simulink model "HQEV_MiL_20160830_integrate"  (Simulink 8.3)
settings: Solver=FixedStepDiscrete  StartTime=0.0  StopTime=inf  FixedStep=0.01  RelTol=1e-3
PostLoadFcn:
  | , if any(exist('dsrtsu_mdlpostloadfcn', 'file') == [2, 3, 6]), try dsrtsu_mdlpostloadfcn('Execute', bdroot); catch fprintf('Error in PostLoadFcn (dsrtsu_mdlpostloadfcn) for model "%s":\n %s\n', bdroot, lasterr); end, end,
values from neighbouring files (symbols this model uses):
  Bat_C_Ah = 36    [parameter_V1.mat]
  Bat_ocv_xIndex = [5 10 20 30 40 50 60 70 80 90 95]    [parameter_V1.mat]
  Bat_ocv_z = [329 332 340 345 347 351 358 372 377 386 391]    [parameter_V1.mat]
  Bat_R_ohm_z = [4.41 3.46 1.57 1.07 0.76 0.63 0.55 0.44 0.41 0.4 0.4 3.14 ... (66 elements, 11x6)]    [parameter_V1.mat]
  Bat_SOC_Init = 90    [parameter_V1.mat]
  Env_hum_pct_Ambient = 30    [parameter_V1.mat]
  Env_Slope_deg = 0    [parameter_V1.mat]
  Env_Temp_degC_Ambient = 25    [parameter_V1.mat]
  Env_v_kmph_HWind = 0    [parameter_V1.mat]
  Reducer_F_i = 7.23    [parameter_V1.mat]
  Reducer_R_i = 7.23    [parameter_V1.mat]
  Veh =     [parameter_V1.mat]
  Veh_A_m2_Fr = 2.246    [parameter_V1.mat]
  Veh_F_Brake =     [parameter_V1.mat]
  Veh_fac_AirDrag = 0.326    [parameter_V1.mat]
  Veh_fac_WhDragFrict_0 = 0.011    [parameter_V1.mat]
  Veh_g_mps2_C = 9.81    [parameter_V1.mat]
  Veh_GainBrake =     [parameter_V1.mat]
  Veh_h_m_COGHigh = 0.5    [parameter_V1.mat]
  Veh_J_kgm2_Wh = 1.3635    [parameter_V1.mat]
  Veh_L_m_AxlBas = 2.63    [parameter_V1.mat]
  Veh_M_kg = 1427    [parameter_V1.mat]
  Veh_mu_Brake = 0.4    [parameter_V1.mat]
  Veh_mu_Tyre =     [parameter_V1.mat]
  Veh_num_FrictPair = 8    [parameter_V1.mat]
  Veh_pct_Brk = 70    [parameter_V1.mat]
  Veh_r_dyn =     [parameter_V1.mat]
  Veh_r_m_BrkDisk = 0.136    [parameter_V1.mat]
  Veh_rho_kgpm3_Air = 1.2258    [parameter_V1.mat]
undefined symbols (not defined in the file or in its folder): DiscIntNeverNeededParam, p_bool_False_M, p_bool_True_M
libraries: BaseOperationLib_Browser x38, simulink x9, DTQC_lib x1, ERR_lib x1, MQM_lib x1, PTCL_lib x1, PUD_lib x1, TQD_lib x1, TQR_lib x1, VMM_lib x1, ACCA_lib x1, BBCA_lib x1
(part 3 of 15)

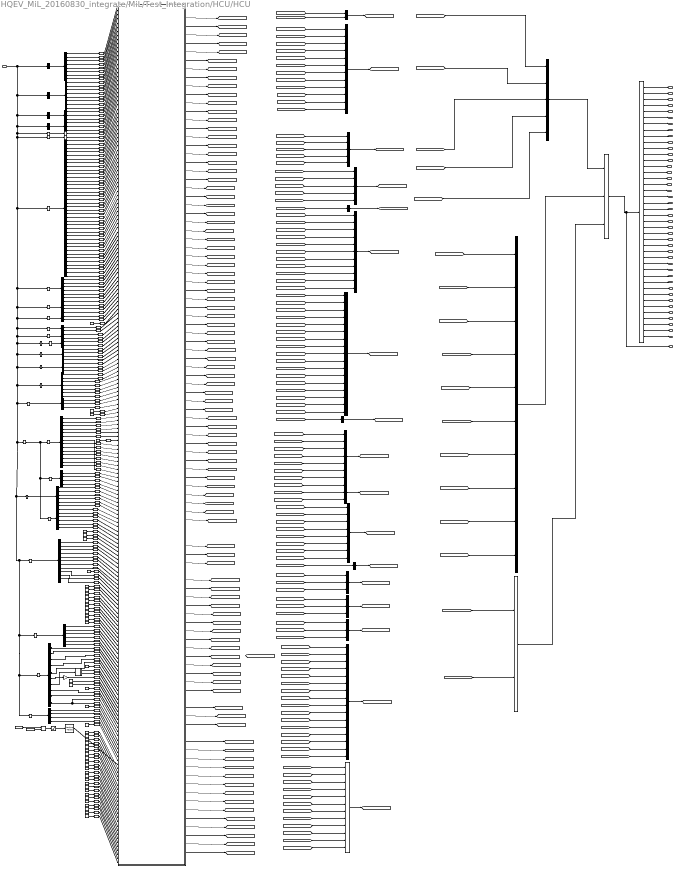
== system HQEV_MiL_20160830_integrate/MiL/Test_Integration/HCU/HCU ==
  In1 : Inport
  AccPedpct2mV : Subsystem
  Bus Creator : BusCreator  Inputs=12
  Bus Creator1 : BusCreator  Inputs=5
  Bus Creator10 : BusCreator  Inputs=8
  Bus Creator11 : BusCreator  Inputs=1
  Bus Creator12 : BusCreator  Inputs=16
  Bus Creator13 : BusCreator  Inputs=12
  Bus Creator{9,14..16,20} (5 alike) : BusCreator  Inputs=3
  Bus Creator17 : BusCreator  Inputs=5
  Bus Creator18 : BusCreator  Inputs=10
  Bus Creator19 : BusCreator  Inputs=2
  Bus Creator2 : BusCreator  Inputs=5
  Bus Creator3 : BusCreator  Inputs=1
  Bus Creator4 : BusCreator  Inputs=2
  Bus Creator5 : BusCreator  Inputs=11
  Bus Creator6 : BusCreator  Inputs=17
  Bus Creator7 : BusCreator  Inputs=1
  Bus Creator8 : BusCreator  Inputs=7
  Bus Selector : BusSelector  OutputSignals=HCU_EVCAN.EV_ACU_1.pOUTP_st_ACU1Crash,HCU_EVCAN.EV_HCU_2.pOUTP_V_HCU2DCDCOutVoltReq,HCU_EVCAN.EV_HCU_2.pOUTP_bool_HCU2DCDCEnbl,HCU_EVCAN.EV_HCU_2.pOUTP_bool_HCU2MainPlusCtrl,HCU_EVCAN.EV_HCU_2.pOUTP_bool_HCU2MainMinusCtrl,HCU_EVCAN.EV_HCU_2.pOUTP_bool_HCU2PreChrgCtrl,HCU_EVCAN.EV_HCU_2.pOUTP_bool_HCU2ChrgPlusCtrl,HCU_EVCAN.EV_HCU_2.pOUTP_bool_HCU2ChrgMinusCtrl,HCU_EVCAN.EV_HCU_2.pOUTP_bool_HCU2SleepIndSig,HCU_EVCAN.EV_HCU_2.pOUTP_st_HCU2ChrgHeatPms,HCU_EVCAN.EV_HCU_2.pOUTP_st_HCU2ChrgConnSt,HCU_EVCAN.EV_HCU_2.pOUTP_bool_HCU2ChrgPms,HCU_EVCAN.EV_HCU_2.pOUTP_st_HCU2VehOprtMode,HCU_EVCAN.EV_HCU_3.pOUTP_Nm_HCU3TMTorqReqToMCU1,HCU_EVCAN.EV_HCU_3.pOUTP_bool_HCU3MotCtlrStModReqToMCU1,HCU_EVCAN.EV_HCU_3.pOUTP_bool_HCU3StopReqToMCU1,HCU_EVCAN.EV_HCU_3.pOUTP_bool_HCU3MotRpdDchaReqToMCU1,HCU_EVCAN.EV_HCU_3.pOUTP_bool_HCU3AntijerkOffReqToMCU1,HCU_EVCAN.EV_HCU_5.pOUTP_Nm_HCU5TMToqReqToMCU2,HCU_EVCAN.EV_HCU_5.pOUTP_bool_HCU5MotCtlrStModReqToMCU2,HCU_EVCAN.EV_HCU_5.pOUTP_bool_HCU5StopReqToMCU2,HCU_EVCAN.EV_HCU_5.pOUTP_bool_HCU5MotRpdDchaReqToMCU2,HCU_EVCAN.EV_HCU_5.pOUTP_bool_HCU5AntijerkOffReqToMCU2,HCU_PTCAN.PT_HCU_13.HCU_VehicleDeiceHeatPermit,HCU_PTCAN.PT_HCU_13.pOUTP_st_HCU13BatPackCoolReq,HCU_PTCAN.PT_HCU_13.pOUTP_bool_HCU13IGOffReq,HCU_PTCAN.PT_HCU_13.HCU_BatterySOCWarning,HCU_PTCAN.PT_HCU_5.pOUTP_st_HCU5EVReady,HCU_PTCAN.PT_HCU_5.pOUTP_st_HCU5HCUStatus,HCU_PTCAN.HCU_Epark.HCU_ParkRequest,HCU_IO.HCU_IO_OUT.pOUTP_pwm_PTCPWMCtrl,HCU_IO.HCU_IO_OUT.pOUTP_bool_LoCoolFanRlyCtrl,HCU_IO.HCU_IO_OUT.pOUTP_bool_HiCoolFanRlyCtrl,HCU_IO.HCU_IO_OUT.pOUTP_pwm_MotWaterPump1Ctrl,HCU_IO.HCU_IO_OUT.pOUTP_pwm_MotWaterPump2Ctrl,HCU_IO.HCU_IO_OUT.pOUTP_pwm_BatWaterPumpCtrl,HCU_PTCAN.PT_HCU_14.HCU_LeverInfo,HCU_PTCAN.PT_HCU_15,HCU_PTCAN.PT_HCU_18,HCU_PTCAN.PT_HCU_19,HCU_PTCAN.PT_HCU_4,HCU_PTCAN.PT_HCU_8
  Bus Selector1 : BusSelector  OutputSignals=MCU_F
  Bus Selector10 : BusSelector  OutputSignals=MCU_F
  Bus Selector11 : BusSelector  OutputSignals=MCU_R
  Bus Selector12 : BusSelector  OutputSignals=MCU2_CoolingRequest
  Bus Selector13 : BusSelector  OutputSignals=BMS
  Bus Selector14 : BusSelector  OutputSignals=BMS_BatteryPackVoltage,BMS_BatteryPackCurrent,BMS_FaultDisposeSignal,BMS_MainPlusContactorCoilState,BMS_MainMinusContactorCoilState,BMS_PrechargeContactorCoilState,BMS_ChargePlusContactorCoilState,BMS_ChargeMinusContactorCoilState,BMS_MainMinusContactorCoilFault,BMS_PrechargeContactorCoilFault,BMS_ChargePlusContactorCoilFault,BMS_ChargeMinusContactorCoilFault,BMS_MainPlusContactorFault,BMS_ChargeRequest,BMS_ChargeStatus,BMS_MainPlusContactorCoilFault,BMS_ChargePlusContactorFault,BMS_BatteryPackStatus,BMS_BatteryChargePowerAvailable_10,BMS_BatteryDischargePowerAvailable_10,BMS_BatteryChargePowerAvailable_2,BMS_BatteryDischargePowerAvailable_2,BMS_BatteryPackSOH,BMS_BatteryPackTemperature,BMS_BatteryPackSOC,BMS_HeatingRequest,BMS_BatteryPackMAXTemperature,BMS_BatteryPackMINTemperature,BMS_BatteryPackInletWaterTemperature,BMS_RemainingEnergyRatio,BMS_ChargeStationOutputCurrent,BMS_ChargeStationOutputVoltage,BMS_InstantPowerConsumption,BMS_ChargeStationStatus,BMS_ChargeStationParameterConfigStatus,BMS_InsulationMonitorWarning,BMS_RemainingChargeTime,BMS_ChargeStationHandShakeStatus
  Bus Selector15 : BusSelector  OutputSignals=DCDC
  Bus Selector16 : BusSelector  OutputSignals=DCDC_OutputCurrent,DCDC_Status,DCDC_OutputVoltage,DCDC_InputCurrent,DCDC_Temperature,DCDC_InputVoltage
  Bus Selector17 : BusSelector  OutputSignals=Charger
  Bus Selector18 : BusSelector  OutputSignals=Charger_Status,Charger_Temperature,Charger_OutputVoltage,Charger_RechargeRequest
  Bus Selector19 : BusSelector  OutputSignals=Airbag
  Bus Selector2 : BusSelector  OutputSignals=MCU1_TMSpeed,MCU1_ActTMTorque,MCU1_TMCapacitanceVoltage,MCU1_ActualTMTorqueValid,MCU1_PrechargeAllow,MCU1_TMStatus,MCU1_TMErrorStatus,MCU1_ShutdownEnable
  Bus Selector20 : BusSelector  OutputSignals=ACU_Crash,ACU_ErrorStatus
  Bus Selector21 : BusSelector  OutputSignals=EPS
  Bus Selector22 : BusSelector  OutputSignals=EPSErrorStatus,SteeringWheelAngleStatus
  Bus Selector23 : BusSelector  OutputSignals=IC
  Bus Selector24 : BusSelector  OutputSignals=HandBrakeSt,DDSPS
  Bus Selector25 : BusSelector  OutputSignals=ESP
  Bus Selector26 : BusSelector  OutputSignals=EPB
  Bus Selector27 : BusSelector  OutputSignals=EPB_Status,EPB_ErrorStatus
  Bus Selector28 : BusSelector  OutputSignals=Epark
  Bus Selector29 : BusSelector  OutputSignals=ParkLock,ParkSensor,DriveSensor,ePARK_CAN_ERR
  Bus Selector3 : BusSelector  OutputSignals=MCU2_TMSpeed,MCU2_ActTMTorque,MCU2_TMCapacitanceVoltage,MCU2_ActualTMTorqueValid,MCU2_PrechargeAllow,MCU2_TMStatus,MCU2_TMErrorStatus,MCUShutdownEnable
  Bus Selector30 : BusSelector  OutputSignals=BCM
  Bus Selector31 : BusSelector  OutputSignals=DriverDoorSt,BCM_HighBeamCmd,WiperStatus
  Bus Selector32 : BusSelector  OutputSignals=Drv
  Bus Selector33 : BusSelector  OutputSignals=signal2.ParkButton (signal 11),signal2.EGSM_ECOSButton (signal 14),signal2.Lever_Position (signal 1)
  Bus Selector34 : BusSelector  OutputSignals=EBS
  Bus Selector35 : BusSelector  OutputSignals=SOC,T_BATT,Status_Temp,ERROR_Calib,Resp_Error,FLAG_INCONSISTENCY,SOC_STATE
  Bus Selector36 : BusSelector  OutputSignals=ESP
  Bus Selector37 : BusSelector  OutputSignals=WheelSpeed_FL,WheelSpeed_FR,ABS_VehicleSpeed,WheelSpeed_RL,WheelSpeed_RR,ABS_MasterCylinderPressure,ABS_ErrorStatus,ABS_Intervention,ASR_ErrorStatus,ASR_Intervention,ESP_ErrorStatus,ESP_Intervention,HHC_Status,HHC_Available
  Bus Selector38 : BusSelector  OutputSignals=ABS
  Bus Selector39 : BusSelector  OutputSignals=YRS
  Bus Selector4 : BusSelector  OutputSignals=MCU_R
  Bus Selector40 : BusSelector  OutputSignals=AX1,AY1,YRSStatus,YRSErrorStatus,AX1Offset,AY1Offset
  Bus Selector41 : BusSelector  OutputSignals=ASR
  Bus Selector42 : BusSelector  OutputSignals=ASR_TorqueReductionFast,MSR_TorqueIncrease,ASR_StatusTRFast,MSR_StatusTI
  Bus Selector43 : BusSelector  OutputSignals=AC
  Bus Selector44 : BusSelector  OutputSignals=AC_CompressorOnRequest,AC_Status,AC_FanRequest,AC_PTCStatus,AC_shutdownEnableL,AC_PowerConsumptionL,AC_PowerConsumptionH,AC_ShutdownEnableH,ACIndication,AC_BLWLevelIndication,AC_OutsideTemperatureIndication
  Bus Selector45 : BusSelector  OutputSignals=ACC
  Bus Selector46 : BusSelector  OutputSignals=ACC_ErrorStatus,ACC_Status,ACC_DecelerationRequest,ACC_StatusTorqueRequest,ACC_TorqueRequest,ACC_StatusACCDecelerationRequest
  Bus Selector47 : BusSelector  OutputSignals=Drv
  Bus Selector48 : BusSelector  OutputSignals=signal2.FastCharge (signal 6),signal2.FastCharge (signal 7),signal2.interlockA (signal 2),signal2.InterlockB (signal 3),signal2.ACC_CruiseButton (signal 16),signal1.AccPed_pct,signal1.BrkPed_pct,signal2.KeyONState (signal 4),signal2.KeyStartState (signal 5),signal1.Brake_OnOff
  Bus Selector49 : BusSelector  OutputSignals=IO
  Bus Selector5 : BusSelector  OutputSignals=MCU1_TM_MAMTorque,MCU1_TM_MAGTorque,MCU1_CalTMTorque
  Bus Selector50 : BusSelector  OutputSignals=SlowChrgSensr1Temp,FastChrgSensr1Temp,SlowChrgSensr2Temp,FastChrgSensr2Temp
  Bus Selector51 : BusSelector  OutputSignals=ESP
  Bus Selector52 : BusSelector  OutputSignals=ASR2.ASR2TrqRdctFastASR2,ASR2.ASR2TrqIncrsMSR2,ASR2.ASR2StTRFastASR2,ASR2.ASR2StTIMSR2,ASR2.ABS6RegenTrqReq,ASR2.ABS6StRegenTrqReq
  Bus Selector6 : BusSelector  OutputSignals=MCU_F
  Bus Selector7 : BusSelector  OutputSignals=MCU_R
  Bus Selector8 : BusSelector  OutputSignals=MCU2_TM_MAMTorque,MCU2_TM_MAGTorque,MCU2_CalTMTorque
  Bus Selector9 : BusSelector  OutputSignals=MCU1_CoolingRequest
  Constant{1..4,6..22,48..68,70,76..77,80} (46 alike) : Constant  Value=0
  Constant23 : Constant  Value=101.325
  Constant24 : Constant
  Constant5 : Constant  Value=2
  Constant73 : Constant  Value=14
  Constant85 : Constant  Value=2
  Data Type Conversion{,1..44,60..80,82,85..105,107..158,160..162,164..167,169..172,177..229,237..241} (209 alike) : DataTypeConversion
  Gain : Gain  Gain=2
  HCU : Subsystem
  Lookup Table : BaseOperationLib_Browser/Lookup Tables Changed/Lookup Table  InputValues=[44.8 44.9 110.2 110.3]  Table=[0 500 4500 4600]  LookUpMeth=Interpolation-Use End Values  OutMin=[]  OutMax=[]  OutDataType=fixdt(1, 16)  OutScaling=2^0  OutDataTypeStr=Inherit: Inherit via back propagation  SaturateOnIntegerOverflow=on
      settings: AttributesFormatString=X:%<InputValues>\nTAB:%<Table>
  Product : Product  RndMeth=Zero
  Saturation : Saturate  UpperLimit=110.3  LowerLimit=44.8
  ACU_Crash : Outport
  HCU_DCDCOutputVoltageRequest : Outport  Port=2
  HCU_DCDCEnable : Outport  Port=3
  HCU_MainPosContactorControl : Outport  Port=4
  HCU_MainNegContactorControl : Outport  Port=5
  HCU_PrechargeContactorControl : Outport  Port=6
  HCU_ChargePosContactorControl : Outport  Port=7
  HCU_ChargeNegContactorControl : Outport  Port=8
  HCU_SleepIndication : Outport  Port=9
  HCU_ChargeHeatingPermission : Outport  Port=10
  HCU_ChargeConnectStatus : Outport  Port=11
  HCU_ChargePermission : Outport  Port=12
  HCU_VehicleOperatingMode : Outport  Port=13
  HCU_TMTorqueRequestToMCU1 : Outport  Port=14
  HCU_StatusTMRequestToMCU1 : Outport  Port=15
  HCU_StopRequestToMCU1 : Outport  Port=16
  HCU_RapidDischargeCmdToMCU1 : Outport  Port=17
  HCU_AntiJerkDisableCmdToMCU1 : Outport  Port=18
  HCU_TMTorqueRequestToMCU2 : Outport  Port=19
  HCU_StatusTMRequestToMCU2 : Outport  Port=20
  HCU_StopRequestToMCU2 : Outport  Port=21
  HCU_RapidDischargeCmdToMCU2 : Outport  Port=22
  HCU_AntiJerkDisableCmdToMCU2 : Outport  Port=23
  HCU_VehicleDeiceHeatPermit : Outport  Port=24
  HCU_BatteryPackCoolRequest : Outport  Port=25
  HCU_IGOFFRequest : Outport  Port=26
  HCU_BatterySOCWarning : Outport  Port=27
  HCU_EVReady : Outport  Port=28
  HCU_Status : Outport  Port=29
  HCU_ParkRequest : Outport  Port=30
  PTC_PWM_pct : Outport  Port=31
  LowSpdFanCmd_na : Outport  Port=32
  HighSpdFanCmd_na : Outport  Port=33
  EM1PumpCmd_pct : Outport  Port=34
  EM2PumpCmd_pct : Outport  Port=35
  BatPumpCmd_pct : Outport  Port=36
  HCU_LeverInfo : Outport  Port=37
  PT_HCU_15 : Outport  Port=38
  PT_HCU_18 : Outport  Port=39
  PT_HCU_19 : Outport  Port=40
  PT_HCU_4 : Outport  Port=41
  PT_HCU_8 : Outport  Port=42
  HCU_Out : Outport  Port=43
  wires:
  [pOUTP_kmph_HCU4VehSpd] -> Bus Creator3/1
  [pOUTP_V_HCU10BatVoltHigh] -> Bus Creator5/1  "pOUTP_V_HCU10BatVoltHigh"
  [pOUTP_st_HCU10ChrgSt] -> Bus Creator5/2  "pOUTP_st_HCU10ChrgSt"
  [pOUTP_A_HCU10BatCurr] -> Bus Creator5/3  "pOUTP_A_HCU10BatCurr"
  [pOUTP_st_HCU10IslaWarning] -> Bus Creator5/4  "pOUTP_st_HCU10IslaWarning"
  [pOUTP_pct_HCU10BatSOC] -> Bus Creator5/5  "pOUTP_pct_HCU10BatSOC"
  [pOUTP_degC_HCU10BatTemp] -> Bus Creator5/6  "pOUTP_degC_HCU10BatTemp"
  [pOUTP_pct_HCU10OutPwr] -> Bus Creator5/7  "pOUTP_pct_HCU10OutPwr"
  [pOUTP_st_HCU10DCDCSt] -> Bus Creator5/8  "pOUTP_st_HCU10DCDCSt"
  [pOUTP_bool_HCU10IntlkSysFlt] -> Bus Creator5/9  "pOUTP_bool_HCU10IntlkSysFlt"
  [pOUTP_bool_HCU10SleepIndSig] -> Bus Creator5/10  "pOUTP_bool_HCU10SleepIndSig"
  [pOUTP_bool_HCU10ECOSwtInd] -> Bus Creator5/11  "pOUTP_bool_HCU10ECOSwtInd"
  [pOUTP_kw_HCU13InstnsPwrCnsmp] -> Bus Creator6/1
  [pOUTP_s_HCU13RemainChrgTime] -> Bus Creator6/2
  [s_RemainDrvgRng_km] -> Bus Creator6/3
  [pOUTP_st_HCU13BatHeatDsply] -> Bus Creator6/4
  [pOUTP_st_HCU13ChrgConnSt] -> Bus Creator6/5
  [pOUTP_bool_HCU13BatErr] -> Bus Creator6/6
  [pOUTP_bool_HCU13TMFlt] -> Bus Creator6/7
  [pOUTP_bool_HCU13TMTempHighAlart] -> Bus Creator6/8
  [pOUTP_st_HCU13IgnKeyPos] -> Bus Creator6/9
  [pOUTP_bool_HCU13ACPTCCnfig] -> Bus Creator6/11
  [s_BatCoolgReq_na] -> Bus Creator6/12
  [HCU_LeverInfo] -> Bus Creator7/1  "HCU_LeverInfo"
  [HCU_CrsCtlSts] -> Bus Creator8/6  "HCU_CrsCtlSts"
  [s_DcDcOutUSp_V] -> Bus Creator/1
  [e_DcDcCmd_na] -> Bus Creator/2
  [s_MaiPosContCmd_na] -> Bus Creator/3
  [s_MaiNegContCmd_na] -> Bus Creator/4
  [s_MaiPrecContCmd_na] -> Bus Creator/5
  [pOUTP_bool_HCU2ChrgPlusCtrl] -> Bus Creator/6
  [pOUTP_bool_HCU2ChrgMinusCtrl] -> Bus Creator/7
  [s_CanSlpCmd_na] -> Bus Creator/8
  [pOUTP_st_HCU2ChrgrHeatReq] -> Bus Creator/9
  [s_ChrgrPlgSwt_na] -> Bus Creator/10
  [s_BatChrgPerm_na] -> Bus Creator/11
  [pOUTP_st_HCU2VehOprtMode] -> Bus Creator/12
  Bus Creator/1 -> [EV_HCU_2]
  [pOUTP_Nm_HCU3TMTorqReqToMCU1] -> Bus Creator1/1  "pOUTP_Nm_HCU3TMTorqReqToMCU1"
  [pOUTP_bool_HCU3MotCtlrStModReqToMCU1] -> Bus Creator1/2  "pOUTP_bool_HCU3MotCtlrStModReqToMCU1"
  [pOUTP_bool_HCU3StopReqToMCU1] -> Bus Creator1/3  "pOUTP_bool_HCU3StopReqToMCU1"
  [pOUTP_bool_HCU3MotRpdDchaReqToMCU1] -> Bus Creator1/4  "pOUTP_bool_HCU3MotRpdDchaReqToMCU1"
  [pOUTP_bool_HCU3AntijerkOffReqToMCU1] -> Bus Creator1/5  "pOUTP_bool_HCU3AntijerkOffReqToMCU1"
  Bus Creator1/1 -> [EV_HCU_3]
  [pOUTP_Nm_HCU5TMToqReqToMCU2] -> Bus Creator2/1  "pOUTP_Nm_HCU5TMToqReqToMCU2"
  [pOUTP_bool_HCU5MotCtlrStModReqToMCU2] -> Bus Creator2/2  "pOUTP_bool_HCU5MotCtlrStModReqToMCU2"
  [pOUTP_bool_HCU5StopReqToMCU2] -> Bus Creator2/3  "pOUTP_bool_HCU5StopReqToMCU2"
  [pOUTP_bool_HCU5MotRpdDchaReqToMCU2] -> Bus Creator2/4  "pOUTP_bool_HCU5MotRpdDchaReqToMCU2"
  [pOUTP_bool_HCU5AntijerkOffReqToMCU2] -> Bus Creator2/5  "pOUTP_bool_HCU5AntijerkOffReqToMCU2"
  Bus Creator4/1 -> [EV_ACU_1]
  Bus Creator2/1 -> [EV_HCU_5]
  Bus Creator3/1 -> [EV_HCU_4]
  Bus Creator5/1 -> [PT_HCU_10]
  [HCU_VehicleDeiceHeatPermit] -> Bus Creator6/10  "HCU_VehicleDeiceHeatPermit"
  [HCU_IGOFFRequest] -> Bus Creator6/13
  [HCU_BatterySOCWarning] -> Bus Creator6/14  "HCU_BatterySOCWarning"
  [HCU_BatteryPackTempWarning] -> Bus Creator6/15  "HCU_BatteryPackTempWarning"
  [HCU_RemainACOnTip] -> Bus Creator6/16  "HCU_RemainACOnTip"
  [HCU_NoiseSimuVoiceConfig] -> Bus Creator6/17  "HCU_NoiseSimuVoiceConfig"
  Bus Creator6/1 -> [PT_HCU_13]
  Bus Creator7/1 -> [PT_HCU_14]
  [HCU_AccPedPosition] -> Bus Creator8/1  "HCU_AccPedPosition"
  [HCU_CalcAccPedPos] -> Bus Creator8/2  "HCU_CalcAccPedPos"
  [HCU_KickdownRequest] -> Bus Creator8/3  "HCU4_KickdownRequest"
  [HCU_BrakeSwitch] -> Bus Creator8/4  "HCU_BrakeSwitch"
  [HCU_ACOnFeedback] -> Bus Creator8/5  "HCU_ACOnFeedback"
  [HCU_AccPedOverride] -> Bus Creator8/7  "HCU4_AccPedOverride"
  Bus Creator8/1 -> [PT_HCU_4]
  [pOUTP_st_HCU5VehOprtMode] -> Bus Creator9/1
  [pOUTP_st_HCU5EVReady] -> Bus Creator9/2
  [pOUTP_st_HCU5HCUStatus] -> Bus Creator9/3
  Bus Creator9/1 -> [PT_HCU_5]
  [HCU_CCMainSwitch] -> Bus Creator10/1  "HCU8_CCMainSwitch"
  [HCU_CCCancelSwitch] -> Bus Creator10/2  "HCU8_CCCancelSwitch"
  [HCU_CCSetOfCoastSwitch] -> Bus Creator10/3  "HCU8_CCSetOfCoastSwitch"
  [HCUCCResumeOrAccSwitch] -> Bus Creator10/4  "HCU8_CCResumeOrAccSwitch"
  [HCU_ResponseACC] -> Bus Creator10/5  "HCU8_ResponseACC"
  [HCU_HeadWaySwitch] -> Bus Creator10/6  "HCU8_HeadWaySwitch"
  [HCU_CCSwitchError] -> Bus Creator10/7  "HCU8_CCSwitchError"
  [HCU_CCTargetSpeed] -> Bus Creator10/8  "HCU_CCTargetSpeed"
  Bus Creator10/1 -> [PT_HCU_8]
  [HCU_ParkRequest] -> Bus Creator11/1  "HCU_ParkRequest"
  Bus Creator11/1 -> [HCU_Epark]
  [pOUTP_bool_MCUEmgnCtrl] -> Bus Creator12/1
  [pOUTP_bool_BMSEmgnCtrl] -> Bus Creator12/2
  [s_PtcCtrlCmd_p100] -> Bus Creator12/3
  [pOUTP_bool_RadorValveCtrlB] -> Bus Creator12/4
  [pOUTP_bool_RadorValveCtrlC] -> Bus Creator12/5
  [pOUTP_bool_BatPTCValveCtrlB] -> Bus Creator12/6
  [pOUTP_bool_BatPTCValveCtrlC] -> Bus Creator12/7
  [s_BrkVacPmpCmd_p100] -> Bus Creator12/8
  [s_LoSpdFanCmd_na] -> Bus Creator12/9
  [s_HiSpdFanCmd_na] -> Bus Creator12/10
  [s_MotWtrPmpCmd_p100] -> Bus Creator12/11
  [s_BatWtrPmpCmd_p100] -> Bus Creator12/12
  [s_MotVirtIgOn_na] -> Bus Creator12/13
  [s_MaiRlyCtlCmd_na] -> Bus Creator12/14
  [pOUTP_bool_VCUSleep] -> Bus Creator12/15
  [IO_Mot2WtrPmpCmd] -> Bus Creator12/16
  Bus Creator12/1 -> [HCU_IO_OUT]
  [s_AccrPedlFlt_na] -> Bus Creator13/1
  [s_MotCtlrFlt_na] -> Bus Creator13/2
  [s_BrkPedlFlt_na] -> Bus Creator13/3
  [s_ThermMngFlt_na] -> Bus Creator13/4
  [s_BmsFlt_na] -> Bus Creator13/5
  [s_VacPmpFlt_na] -> Bus Creator13/6
  [s_BMSIFlt_na] -> Bus Creator13/7
  [s_ChrgrFlt_na] -> Bus Creator13/8
  [s_EspFlt_na] -> Bus Creator13/9
  [s_CrcCtlFlt_na] -> Bus Creator13/10
  [s_DcDcFlt_na] -> Bus Creator13/11
  [s_IgFlt_na] -> Bus Creator13/12
  Bus Creator13/1 -> [HCU_Fault_OUT]
  [pOUTP_kmph_ABS1VehSpd] -> Bus Creator4/1
  [pOUTP_st_Airbag1CrashIntsy] -> Bus Creator4/2
  [EV_ACU_1] -> Bus Creator17/1  "EV_ACU_1"
  [EV_HCU_2] -> Bus Creator17/2  "EV_HCU_2"
  [EV_HCU_3] -> Bus Creator17/3  "EV_HCU_3"
  [EV_HCU_4] -> Bus Creator17/4  "EV_HCU_4"
  [EV_HCU_5] -> Bus Creator17/5  "EV_HCU_5"
  [PT_HCU_10] -> Bus Creator18/1  "PT_HCU_10"
  [PT_HCU_13] -> Bus Creator18/2  "PT_HCU_13"
  [PT_HCU_14] -> Bus Creator18/3  "PT_HCU_14"
  [PT_HCU_4] -> Bus Creator18/4  "PT_HCU_4"
  [PT_HCU_5] -> Bus Creator18/5  "PT_HCU_5"
  [PT_HCU_8] -> Bus Creator18/6  "PT_HCU_8"
  [HCU_Epark] -> Bus Creator18/7  "HCU_Epark"
  [HCU_IO_OUT] -> Bus Creator19/1  "HCU_IO_OUT"
  [HCU_Fault_OUT] -> Bus Creator19/2  "HCU_Fault_OUT"
  Bus Creator17/1 -> Bus Creator16/1  "HCU_EVCAN"
  Bus Creator18/1 -> Bus Creator16/2  "HCU_PTCAN"
  Bus Creator19/1 -> Bus Creator16/3  "HCU_IO"
  Bus Creator16/1 -> HCU_Out/1, Bus Selector/1
  Bus Selector/1 -> ACU_Crash/1  "<pOUTP_st_ACU1Crash>"
  Bus Selector/2 -> HCU_DCDCOutputVoltageRequest/1  "<pOUTP_V_HCU2DCDCOutVoltReq>"
  Bus Selector/3 -> HCU_DCDCEnable/1  "<pOUTP_bool_HCU2DCDCEnbl>"
  Bus Selector/4 -> HCU_MainPosContactorControl/1  "<pOUTP_bool_HCU2MainPlusCtrl>"
  Bus Selector/7 -> HCU_ChargePosContactorControl/1  "<pOUTP_bool_HCU2ChrgPlusCtrl>"
  Bus Selector/8 -> HCU_ChargeNegContactorControl/1  "<pOUTP_bool_HCU2ChrgMinusCtrl>"
  Bus Selector/9 -> HCU_SleepIndication/1  "<pOUTP_bool_HCU2SleepIndSig>"
  Bus Selector/10 -> HCU_ChargeHeatingPermission/1  "<pOUTP_st_HCU2ChrgHeatPms>"
  Bus Selector/11 -> HCU_ChargeConnectStatus/1  "<pOUTP_st_HCU2ChrgConnSt>"
  Bus Selector/12 -> HCU_ChargePermission/1  "<pOUTP_bool_HCU2ChrgPms>"
  Bus Selector/13 -> HCU_VehicleOperatingMode/1  "<pOUTP_st_HCU2VehOprtMode>"
  Bus Selector/14 -> HCU_TMTorqueRequestToMCU1/1  "<pOUTP_Nm_HCU3TMTorqReqToMCU1>"
  Bus Selector/15 -> HCU_StatusTMRequestToMCU1/1  "<pOUTP_bool_HCU3MotCtlrStModReqToMCU1>"
  Bus Selector/16 -> HCU_StopRequestToMCU1/1  "<pOUTP_bool_HCU3StopReqToMCU1>"
  Bus Selector/17 -> HCU_RapidDischargeCmdToMCU1/1  "<pOUTP_bool_HCU3MotRpdDchaReqToMCU1>"
  Bus Selector/18 -> HCU_AntiJerkDisableCmdToMCU1/1  "<pOUTP_bool_HCU3AntijerkOffReqToMCU1>"
  Bus Selector/19 -> HCU_TMTorqueRequestToMCU2/1  "<pOUTP_Nm_HCU5TMToqReqToMCU2>"
  Bus Selector/20 -> HCU_StatusTMRequestToMCU2/1  "<pOUTP_bool_HCU5MotCtlrStModReqToMCU2>"
  Bus Selector/21 -> HCU_StopRequestToMCU2/1  "<pOUTP_bool_HCU5StopReqToMCU2>"
  Bus Selector/22 -> HCU_RapidDischargeCmdToMCU2/1  "<pOUTP_bool_HCU5MotRpdDchaReqToMCU2>"
  Bus Selector/23 -> HCU_AntiJerkDisableCmdToMCU2/1  "<pOUTP_bool_HCU5AntijerkOffReqToMCU2>"
  Bus Selector/24 -> HCU_VehicleDeiceHeatPermit/1  "<HCU_VehicleDeiceHeatPermit>"
  Bus Selector/25 -> HCU_BatteryPackCoolRequest/1  "<pOUTP_st_HCU13BatPackCoolReq>"
  Bus Selector/26 -> HCU_IGOFFRequest/1  "<pOUTP_bool_HCU13IGOffReq>"
  Bus Selector/27 -> HCU_BatterySOCWarning/1  "<HCU_BatterySOCWarning>"
  Bus Selector/28 -> HCU_EVReady/1  "<pOUTP_st_HCU5EVReady>"
  Bus Selector/29 -> HCU_Status/1  "<pOUTP_st_HCU5HCUStatus>"
  Bus Selector/30 -> HCU_ParkRequest/1  "<HCU_ParkRequest>"
  Bus Selector/32 -> LowSpdFanCmd_na/1  "<pOUTP_bool_LoCoolFanRlyCtrl>"
  Bus Selector/33 -> HighSpdFanCmd_na/1  "<pOUTP_bool_HiCoolFanRlyCtrl>"
  Bus Selector/31 -> PTC_PWM_pct/1  "<pOUTP_pwm_PTCPWMCtrl>"
  Bus Selector/34 -> EM1PumpCmd_pct/1  "<pOUTP_pwm_MotWaterPump1Ctrl>"
  Bus Selector/35 -> EM2PumpCmd_pct/1  "<pOUTP_pwm_MotWaterPump2Ctrl>"
  Bus Selector/36 -> BatPumpCmd_pct/1  "<pOUTP_pwm_BatWaterPumpCtrl>"
  Bus Selector1/1 -> Bus Selector2/1  "<MCU_F>"
  Bus Selector2/1 -> Data Type Conversion153/1  "<MCU1_TMSpeed>"
  Bus Selector2/2 -> Data Type Conversion150/1  "<MCU1_ActTMTorque>"
  Bus Selector2/3 -> Data Type Conversion152/1  "<MCU1_TMCapacitanceVoltage>"
  Bus Selector2/4 -> Data Type Conversion151/1  "<MCU1_ActualTMTorqueValid>"
  Bus Selector2/5 -> Data Type Conversion149/1  "<MCU1_PrechargeAllow>"
  Bus Selector2/6 -> Data Type Conversion148/1  "<MCU1_TMStatus>"
  Bus Selector2/7 -> Data Type Conversion147/1  "<MCU1_TMErrorStatus>"
  Bus Selector4/1 -> Bus Selector3/1  "<MCU_R>"
  Bus Selector3/1 -> Data Type Conversion146/1  "<MCU2_TMSpeed>"
  Bus Selector3/7 -> Data Type Conversion140/1  "<MCU2_TMErrorStatus>"
  Bus Selector3/5 -> Data Type Conversion142/1  "<MCU2_PrechargeAllow>"
  Bus Selector3/4 -> Data Type Conversion143/1  "<MCU2_ActualTMTorqueValid>"
  Bus Selector3/2 -> Data Type Conversion145/1  "<MCU2_ActTMTorque>"
  Bus Selector3/3 -> Data Type Conversion144/1  "<MCU2_TMCapacitanceVoltage>"
  Bus Selector3/6 -> Data Type Conversion141/1  "<MCU2_TMStatus>"
  Bus Selector6/1 -> Bus Selector5/1  "<MCU_F>"
  Bus Selector5/1 -> Data Type Conversion139/1  "<MCU1_TM_MAMTorque>"
  Bus Selector5/2 -> Data Type Conversion136/1  "<MCU1_TM_MAGTorque>"
  Bus Selector5/3 -> Data Type Conversion138/1  "<MCU1_CalTMTorque>"
  Bus Selector7/1 -> Bus Selector8/1  "<MCU_R>"
  Bus Selector8/2 -> Data Type Conversion135/1  "<MCU2_TM_MAGTorque>"
  Bus Selector8/1 -> Data Type Conversion137/1  "<MCU2_TM_MAMTorque>"
  Bus Selector8/3 -> Data Type Conversion134/1  "<MCU2_CalTMTorque>"
  Bus Selector10/1 -> Bus Selector9/1  "<MCU_F>"
  Bus Selector9/1 -> Data Type Conversion133/1  "<MCU1_CoolingRequest>"
  Bus Selector11/1 -> Bus Selector12/1  "<MCU_R>"
  Bus Selector12/1 -> Data Type Conversion132/1  "<MCU2_CoolingRequest>"
  Bus Selector13/1 -> Bus Selector14/1  "<BMS>"
  Bus Selector14/1 -> Data Type Conversion131/1  "<BMS_BatteryPackVoltage>"
  Bus Selector14/2 -> Data Type Conversion130/1  "<BMS_BatteryPackCurrent>"
  Bus Selector14/3 -> Data Type Conversion129/1  "<BMS_FaultDisposeSignal>"
  Bus Selector14/4 -> Data Type Conversion128/1  "<BMS_MainPlusContactorCoilState>"
  Bus Selector14/5 -> Data Type Conversion127/1  "<BMS_MainMinusContactorCoilState>"
  Bus Selector14/6 -> Data Type Conversion126/1  "<BMS_PrechargeContactorCoilState>"
  Bus Selector14/7 -> Data Type Conversion125/1  "<BMS_ChargePlusContactorCoilState>"
  Bus Selector14/8 -> Data Type Conversion122/1  "<BMS_ChargeMinusContactorCoilState>"
  Bus Selector14/9 -> Data Type Conversion124/1  "<BMS_MainMinusContactorCoilFault>"
  Bus Selector14/10 -> Data Type Conversion123/1  "<BMS_PrechargeContactorCoilFault>"
  Bus Selector14/11 -> Data Type Conversion121/1  "<BMS_ChargePlusContactorCoilFault>"
  Bus Selector14/12 -> Data Type Conversion120/1  "<BMS_ChargeMinusContactorCoilFault>"
  Bus Selector14/13 -> Data Type Conversion119/1  "<BMS_MainPlusContactorFault>"
  Bus Selector14/14 -> Data Type Conversion118/1  "<BMS_ChargeRequest>"
  Bus Selector14/15 -> Data Type Conversion117/1  "<BMS_ChargeStatus>"
  Bus Selector14/16 -> Data Type Conversion116/1  "<BMS_MainPlusContactorCoilFault>"
  Bus Selector14/17 -> Data Type Conversion115/1  "<BMS_ChargePlusContactorFault>"
  Bus Selector14/18 -> Data Type Conversion114/1  "<BMS_BatteryPackStatus>"
  Bus Selector14/19 -> Data Type Conversion113/1  "<BMS_BatteryChargePowerAvailable_10>"
  Bus Selector14/20 -> Data Type Conversion112/1  "<BMS_BatteryDischargePowerAvailable_10>"
  Bus Selector14/21 -> Data Type Conversion111/1  "<BMS_BatteryChargePowerAvailable_2>"
  Bus Selector14/22 -> Data Type Conversion108/1  "<BMS_BatteryDischargePowerAvailable_2>"
  Bus Selector14/23 -> Data Type Conversion110/1  "<BMS_BatteryPackSOH>"
  Bus Selector14/24 -> Data Type Conversion109/1  "<BMS_BatteryPackTemperature>"
  Bus Selector14/25 -> Data Type Conversion95/1  "<BMS_BatteryPackSOC>"
  Bus Selector14/27 -> Data Type Conversion93/1  "<BMS_BatteryPackMAXTemperature>"
  Bus Selector14/29 -> Data Type Conversion91/1  "<BMS_BatteryPackInletWaterTemperature>"
  Bus Selector14/28 -> Data Type Conversion92/1  "<BMS_BatteryPackMINTemperature>"
  Bus Selector14/26 -> Data Type Conversion94/1  "<BMS_HeatingRequest>"
  Bus Selector14/30 -> Data Type Conversion90/1  "<BMS_RemainingEnergyRatio>"
  Bus Selector14/31 -> Data Type Conversion89/1  "<BMS_ChargeStationOutputCurrent>"
  Bus Selector14/32 -> Data Type Conversion88/1  "<BMS_ChargeStationOutputVoltage>"
  Bus Selector14/33 -> Data Type Conversion87/1  "<BMS_InstantPowerConsumption>"
  Bus Selector14/34 -> Data Type Conversion86/1  "<BMS_ChargeStationStatus>"
  Bus Selector14/35 -> Data Type Conversion85/1  "<BMS_ChargeStationParameterConfigStatus>"
  Bus Selector14/37 -> Data Type Conversion107/1  "<BMS_RemainingChargeTime>"
  Bus Selector14/38 -> Data Type Conversion32/1  "<BMS_ChargeStationHandShakeStatus>"
  Bus Selector15/1 -> Bus Selector16/1  "<DCDC>"
  Bus Selector14/36 -> Data Type Conversion/1  "<BMS_InsulationMonitorWarning>"
  Bus Selector16/1 -> Data Type Conversion105/1  "<DCDC_OutputCurrent>"
  Bus Selector16/2 -> Data Type Conversion104/1  "<DCDC_Status>"
  Bus Selector16/3 -> Data Type Conversion103/1  "<DCDC_OutputVoltage>"
  Bus Selector16/4 -> Data Type Conversion102/1  "<DCDC_InputCurrent>"
  Bus Selector16/5 -> Data Type Conversion101/1  "<DCDC_Temperature>"
  Bus Selector16/6 -> Data Type Conversion100/1  "<DCDC_InputVoltage>"
  Bus Selector17/1 -> Bus Selector18/1  "<Charger>"
  Bus Selector18/1 -> Data Type Conversion99/1  "<Charger_Status>"
  Bus Selector18/2 -> Data Type Conversion98/1  "<Charger_Temperature>"
  Bus Selector18/3 -> Data Type Conversion97/1  "<Charger_OutputVoltage>"
  Bus Selector18/4 -> Data Type Conversion96/1  "<Charger_RechargeRequest>"
  Bus Selector19/1 -> Bus Selector20/1  "<Airbag>"
  Bus Selector20/1 -> Data Type Conversion158/1  "<ACU_Crash>"
  Bus Selector20/2 -> Data Type Conversion157/1  "<ACU_ErrorStatus>"
  Bus Selector21/1 -> Bus Selector22/1  "<EPS>"
  Bus Selector22/2 -> Data Type Conversion155/1  "<SteeringWheelAngleStatus>"
  Bus Selector22/1 -> Data Type Conversion156/1  "<EPSErrorStatus>"
  Bus Selector23/1 -> Bus Selector24/1  "<IC>"
  Bus Selector24/2 -> Data Type Conversion162/1  "<DDSPS>"
  Bus Selector24/1 -> Data Type Conversion154/1  "<HandBrakeSt>"
  Bus Selector25/1 -> Bus Selector26/1  "<ESP>"
  Bus Selector26/1 -> Bus Selector27/1  "<EPB>"
  Bus Selector27/1 -> Data Type Conversion161/1  "<EPB_Status>"
  Bus Selector27/2 -> Data Type Conversion160/1  "<EPB_ErrorStatus>"
  Bus Selector28/1 -> Bus Selector29/1  "<Epark>"
  Bus Selector29/1 -> Data Type Conversion167/1  "<ParkLock>"
  Bus Selector29/2 -> Data Type Conversion166/1  "<ParkSensor>"
  Bus Selector29/3 -> Data Type Conversion165/1  "<DriveSensor>"
  Bus Selector30/1 -> Bus Selector31/1  "<BCM>"
  Bus Selector31/2 -> Data Type Conversion172/1  "<BCM_HighBeamCmd>"
  Bus Selector31/3 -> Data Type Conversion171/1  "<WiperStatus>"
  Bus Selector31/1 -> Data Type Conversion164/1  "<DriverDoorSt>"
  Bus Selector32/1 -> Bus Selector33/1  "<Drv>"
  Bus Selector33/1 -> Data Type Conversion182/1  "<ParkButton (signal 11)>"
  Bus Selector33/2 -> Data Type Conversion181/1  "<EGSM_ECOSButton (signal 14)>"
  Bus Selector33/3 -> Data Type Conversion180/1  "<Lever_Position (signal 1)>"
  Bus Selector34/1 -> Bus Selector35/1  "<EBS>"
  Bus Selector35/2 -> Data Type Conversion169/1  "<T_BATT>"
  Bus Selector35/1 -> Data Type Conversion170/1  "<SOC>"
  Bus Selector35/3 -> Data Type Conversion177/1  "<Status_Temp>"
  Bus Selector35/4 -> Data Type Conversion190/1  "<ERROR_Calib>"
  Bus Selector35/5 -> Data Type Conversion189/1  "<Resp_Error>"
  Bus Selector35/6 -> Data Type Conversion188/1  "<FLAG_INCONSISTENCY>"
  Bus Selector35/7 -> Data Type Conversion187/1  "<SOC_STATE>"
  Bus Selector36/1 -> Bus Selector38/1, Bus Selector39/1, Bus Selector41/1  "<ESP>"
  Bus Selector38/1 -> Bus Selector37/1  "<ABS>"
  Bus Selector37/1 -> Data Type Conversion179/1  "<WheelSpeed_FL>"
  Bus Selector37/2 -> Data Type Conversion178/1  "<WheelSpeed_FR>"
  Bus Selector37/3 -> Data Type Conversion186/1  "<ABS_VehicleSpeed>"
  Bus Selector37/4 -> Data Type Conversion185/1  "<WheelSpeed_RL>"
  Bus Selector37/5 -> Data Type Conversion184/1  "<WheelSpeed_RR>"
  Bus Selector37/6 -> Data Type Conversion183/1  "<ABS_MasterCylinderPressure>"
  Bus Selector37/7 -> Data Type Conversion191/1  "<ABS_ErrorStatus>"
  Bus Selector37/8 -> Data Type Conversion204/1  "<ABS_Intervention>"
  Bus Selector37/9 -> Data Type Conversion203/1  "<ASR_ErrorStatus>"
  Bus Selector37/10 -> Data Type Conversion202/1  "<ASR_Intervention>"
  Bus Selector37/11 -> Data Type Conversion201/1  "<ESP_ErrorStatus>"
  Bus Selector37/12 -> Data Type Conversion196/1  "<ESP_Intervention>"
  Bus Selector37/13 -> Data Type Conversion195/1  "<HHC_Status>"
  Bus Selector37/14 -> Data Type Conversion194/1  "<HHC_Available>"
  Bus Selector40/1 -> Data Type Conversion206/1  "<AX1>"
  Bus Selector40/2 -> Data Type Conversion205/1  "<AY1>"
  Bus Selector40/3 -> Data Type Conversion193/1  "<YRSStatus>"
  Bus Selector40/4 -> Data Type Conversion192/1  "<YRSErrorStatus>"
  Bus Selector40/5 -> Data Type Conversion208/1  "<AX1Offset>"
  Bus Selector40/6 -> Data Type Conversion207/1  "<AY1Offset>"
  Bus Selector41/1 -> Bus Selector42/1  "<ASR>"
  Bus Selector42/1 -> Data Type Conversion200/1  "<ASR_TorqueReductionFast>"
  Bus Selector42/2 -> Data Type Conversion199/1  "<MSR_TorqueIncrease>"
  Bus Selector42/3 -> Data Type Conversion198/1  "<ASR_StatusTRFast>"
  Bus Selector42/4 -> Data Type Conversion197/1  "<MSR_StatusTI>"
  Bus Selector43/1 -> Bus Selector44/1  "<AC>"
  Bus Selector44/1 -> Data Type Conversion209/1  "<AC_CompressorOnRequest>"
  Bus Selector44/2 -> Data Type Conversion210/1  "<AC_Status>"
  Bus Selector44/3 -> Data Type Conversion211/1  "<AC_FanRequest>"
  Bus Selector44/4 -> Data Type Conversion212/1  "<AC_PTCStatus>"
  Bus Selector44/5 -> Data Type Conversion213/1  "<AC_shutdownEnableL>"
  Bus Selector44/6 -> Data Type Conversion214/1  "<AC_PowerConsumptionL>"
  Bus Selector44/7 -> Data Type Conversion215/1  "<AC_PowerConsumptionH>"
  Bus Selector44/8 -> Data Type Conversion216/1  "<AC_ShutdownEnableH>"
  Bus Selector44/9 -> Data Type Conversion217/1  "<ACIndication>"
  Bus Selector44/10 -> Data Type Conversion218/1  "<AC_BLWLevelIndication>"
  Constant1/1 -> Data Type Conversion3/1
  Constant2/1 -> Data Type Conversion4/1
  Constant3/1 -> Data Type Conversion5/1
  Constant4/1 -> Data Type Conversion6/1
  Constant8/1 -> Data Type Conversion9/1
  Constant6/1 -> Data Type Conversion7/1
  Constant7/1 -> Data Type Conversion8/1
  Constant11/1 -> Data Type Conversion10/1
  Constant14/1 -> Data Type Conversion13/1
  Constant12/1 -> Data Type Conversion11/1
  Constant13/1 -> Data Type Conversion12/1
  Constant18/1 -> Data Type Conversion16/1
  Constant16/1 -> Data Type Conversion14/1
  Constant17/1 -> Data Type Conversion15/1
  Constant20/1 -> Data Type Conversion17/1
  Bus Selector45/1 -> Bus Selector46/1  "<ACC>"
  Bus Selector46/1 -> Data Type Conversion228/1  "<ACC_ErrorStatus>"
  Bus Selector46/2 -> Data Type Conversion220/1  "<ACC_Status>"
  Bus Selector46/3 -> Data Type Conversion221/1  "<ACC_DecelerationRequest>"
  Bus Selector46/4 -> Data Type Conversion222/1  "<ACC_StatusTorqueRequest>"
  Bus Selector46/5 -> Data Type Conversion223/1  "<ACC_TorqueRequest>"
  Bus Selector46/6 -> Data Type Conversion224/1  "<ACC_StatusACCDecelerationRequest>"
  Constant21/1 -> Data Type Conversion34/1
  Constant22/1 -> Data Type Conversion33/1
  Constant48/1 -> Data Type Conversion60/1
  Constant49/1 -> Data Type Conversion61/1
  Constant50/1 -> Data Type Conversion62/1
  Constant51/1 -> Data Type Conversion63/1
  Constant52/1 -> Data Type Conversion64/1
  Constant53/1 -> Data Type Conversion65/1
  Constant54/1 -> Data Type Conversion66/1
  Constant55/1 -> Data Type Conversion67/1
  Constant56/1 -> Data Type Conversion68/1
  Constant57/1 -> Data Type Conversion69/1
  Constant58/1 -> Data Type Conversion70/1
  Constant59/1 -> Data Type Conversion71/1
  Constant60/1 -> Data Type Conversion72/1
  Constant61/1 -> Data Type Conversion73/1
  Constant62/1 -> Data Type Conversion74/1
  Constant63/1 -> Data Type Conversion75/1
  Constant64/1 -> Data Type Conversion76/1
  Constant65/1 -> Data Type Conversion77/1
  Constant66/1 -> Data Type Conversion78/1
  Constant67/1 -> Data Type Conversion79/1
  Constant68/1 -> Data Type Conversion80/1
  Constant70/1 -> Data Type Conversion82/1
  Bus Selector47/1 -> Bus Selector48/1  "<Drv>"
  Bus Selector48/1 -> Data Type Conversion225/1  "<FastCharge (signal 6)>"
  Bus Selector48/2 -> Data Type Conversion226/1  "<FastCharge (signal 7)>"
  Bus Selector44/11 -> Data Type Conversion219/1  "<AC_OutsideTemperatureIndication>"
  Constant5/1 -> Data Type Conversion24/1
  Constant76/1 -> Data Type Conversion25/1
  Constant77/1 -> Data Type Conversion30/1
  AccPedpct2mV/1(Out1) -> Data Type Conversion20/1
  Constant80/1 -> Data Type Conversion19/1
  Bus Selector48/5 -> Data Type Conversion18/1  "<ACC_CruiseButton (signal 16)>"
  Bus Selector48/9 -> Data Type Conversion27/1  "<KeyStartState (signal 5)>"
  AccPedpct2mV/2(Out2) -> Data Type Conversion21/1
  Bus Selector48/6 -> AccPedpct2mV/1(In1)  "<AccPed_pct>"
  Constant73/1 -> Data Type Conversion23/1
  Bus Selector48/8 -> Data Type Conversion26/1  "<KeyONState (signal 4)>"
  Bus Selector48/7 -> Gain/1  "<BrkPed_pct>"
  Bus Selector48/10 -> Data Type Conversion28/1, Data Type Conversion29/1  "<Brake_OnOff>"
  Gain/1 -> Data Type Conversion22/1
  Bus Selector/6 -> HCU_PrechargeContactorControl/1  "<pOUTP_bool_HCU2PreChrgCtrl>"
  Bus Selector/5 -> HCU_MainNegContactorControl/1  "<pOUTP_bool_HCU2MainMinusCtrl>"
  Data Type Conversion139/1 -> HCU/17(pCANR_Nm_MCU12TMMAMTrq)
  Data Type Conversion136/1 -> HCU/18(pCANR_Nm_MCU12TMMAGTrq)
  Data Type Conversion138/1 -> HCU/19(pCANR_Nm_MCU12CalTMTrq)
  Data Type Conversion137/1 -> HCU/20(pCANR_Nm_MCU22TMMAMTrq)
  Data Type Conversion135/1 -> HCU/21(pCANR_Nm_MCU22TMMAGTrq)
  Data Type Conversion134/1 -> HCU/22(pCANR_Nm_MCU22CalTMTrq)
  Data Type Conversion133/1 -> HCU/23(pCANR_st_MCU13CoolReq)
  Data Type Conversion132/1 -> HCU/24(pCANR_st_MCU23CoolReq)
  Data Type Conversion131/1 -> HCU/25(pCANR_V_BMS1BatPackVolt)
  Data Type Conversion130/1 -> HCU/26(pCANR_A_BMS1BatPackCurr)
  Data Type Conversion129/1 -> HCU/27(pCANR_bool_BMS1FltDisposeSig)
  Data Type Conversion128/1 -> HCU/28(pCANR_bool_BMS1MainPlusCoilSt)
  Data Type Conversion127/1 -> HCU/29(pCANR_bool_BMS1MainMinusCoilSt)
  Data Type Conversion126/1 -> HCU/30(pCANR_bool_BMS1PreChrgCoilSt)
  Data Type Conversion125/1 -> HCU/31(pCANR_bool_BMS1ChrgPlusCoilSt)
  Data Type Conversion122/1 -> HCU/32(pCANR_bool_BMS1ChrgMinusCoilSt)
  Data Type Conversion124/1 -> HCU/33(pCANR_st_BMS1MainMinusCoilFlt)
  Data Type Conversion123/1 -> HCU/34(pCANR_st_BMS1PrechrgCoilFlt)
  Data Type Conversion121/1 -> HCU/35(pCANR_st_BMS1ChrgPlusCoilFlt)
  Data Type Conversion120/1 -> HCU/36(pCANR_st_BMS1ChrgMinusCoilFlt)
  Data Type Conversion119/1 -> HCU/37(pCANR_st_BMS1MainPlusFlt)
  Data Type Conversion118/1 -> HCU/38(pCANR_bool_BMS1ChrgReq)
  Data Type Conversion117/1 -> HCU/39(pCANR_st_BMS1ChrgSt)
  Data Type Conversion116/1 -> HCU/40(pCANR_st_BMS1ChrgPlusFlt)
  Data Type Conversion115/1 -> HCU/41(pCANR_st_BMS1MainPlusCoilFlt)
  Data Type Conversion114/1 -> HCU/42(pCANR_st_BMS1BatPackSt)
  Data Type Conversion113/1 -> HCU/43(pCANR_kw_BMS2ChrgPwrAvail10)
  Data Type Conversion112/1 -> HCU/44(pCANR_kw_BMS2DischrgPwrAvail10)
  Data Type Conversion111/1 -> HCU/45(pCANR_kw_BMS2ChrgPwrAvail2)
  Data Type Conversion108/1 -> HCU/46(pCANR_kw_BMS2DischrgPwrAvail2)
  Data Type Conversion110/1 -> HCU/47(pCANR_pct_BMS3BatPackSOH)
  Data Type Conversion109/1 -> HCU/48(pCANR_degC_BMS3BatPackTemp)
  Data Type Conversion95/1 -> HCU/49(pCANR_pct_BMS3BatPackSOC)
  Data Type Conversion94/1 -> HCU/50(pCANR_bool_BMS3HeatReq)
  Data Type Conversion93/1 -> HCU/51(pCANR_degC_BMS5BatMaxTemp)
  Data Type Conversion92/1 -> HCU/52(pCANR_degC_BMS5BatMinTemp)
  Data Type Conversion91/1 -> HCU/53(pCANR_degC_BMS5BatInWaterTemp)
  Data Type Conversion90/1 -> HCU/54(pCANR_pct_BMS5RemainEngyRatio)
  Data Type Conversion89/1 -> HCU/55(pCANR_A_BMS6ChrgStationOutCurr)
  Data Type Conversion88/1 -> HCU/56(pCANR_V_BMS6ChrgStationOutVolt)
  Data Type Conversion87/1 -> HCU/57(pCANR_kw_BMS6InstnsPwrCnsmp)
  Data Type Conversion86/1 -> HCU/58(pCANR_st_BMS5ChrgStationSt)
  Data Type Conversion85/1 -> HCU/59(pCANR_st_BMS6ChrgStationCnfigSt)
  Data Type Conversion/1 -> HCU/60(pCANR_st_BMS5IslaWarning)
  Data Type Conversion107/1 -> HCU/61(pCANR_min_BMS5RemainChrgTime)
  Data Type Conversion105/1 -> HCU/63(pCANR_A_DCDC1OutCurr)
  Data Type Conversion104/1 -> HCU/64(pCANR_st_DCDC1St)
  Data Type Conversion103/1 -> HCU/65(pCANR_V_DCDC1COutVolt)
  Data Type Conversion102/1 -> HCU/66(pCANR_A_DCDC1InCurr)
  Data Type Conversion101/1 -> HCU/67(pCANR_degC_DCDC1Temp)
  Data Type Conversion100/1 -> HCU/68(pCANR_V_DCDC1InVolt)
  Data Type Conversion99/1 -> HCU/69(pCANR_st_Charger1ChrgrSt)
  Data Type Conversion98/1 -> HCU/70(pCANR_degC_Charger1ChrgrTemp)
  Data Type Conversion97/1 -> HCU/71(pCANR_V_Charger1ChrgrOutVolt)
  Data Type Conversion96/1 -> HCU/72(pCANR_bool_Charger1RechrgReq)
  Data Type Conversion158/1 -> HCU/73(pCANR_st_ACU1Crash)
  Data Type Conversion157/1 -> HCU/74(pCANR_st_ACU1ErrSt)
  Data Type Conversion155/1 -> HCU/77(pCANR_st_SAS1SASSt)
  Data Type Conversion154/1 -> HCU/78(pCANR_st_IC1HandBrkSt)
  Data Type Conversion162/1 -> HCU/79(pCANR_km_IC2DDSPS)
  Data Type Conversion161/1 -> HCU/80(pCANR_st_EPB1EPBSt)
  Data Type Conversion160/1 -> HCU/81(pCANR_bool_EPB1EPBErrSt)
  Data Type Conversion167/1 -> HCU/82(pCANR_st_EparkPrkLock)
  Data Type Conversion166/1 -> HCU/83(pCANR_bool_EparkPrkSensor)
  Data Type Conversion165/1 -> HCU/84(pCANR_bool_EparkDrvSensor)
  Data Type Conversion164/1 -> HCU/86(pCANR_bool_BCM13DrvDoorSt)
  Data Type Conversion172/1 -> HCU/87(pCANR_bool_BCM13HighBeamCmd)
  Data Type Conversion171/1 -> HCU/88(pCANR_st_BCM13WiperStatus)
  Data Type Conversion170/1 -> HCU/89(pCANR_pct_EEM1SOC)
  Data Type Conversion169/1 -> HCU/90(pCANR_degC_EEM1BATTTemp)
  Data Type Conversion177/1 -> HCU/91(pCANR_st_EEM1TempSt)
  Data Type Conversion190/1 -> HCU/92(pCANR_bool_EEM1CalibError)
  Data Type Conversion189/1 -> HCU/93(pCANR_bool_EEM1RespError)
  Data Type Conversion188/1 -> HCU/94(pCANR_bool_EEM1InconsFlag)
  Data Type Conversion187/1 -> HCU/95(pCANR_st_EEM1SOCSt)
  Data Type Conversion182/1 -> HCU/96(pCANR_st_EGSM1PrkLockBtnSts)
  Data Type Conversion181/1 -> HCU/97(pCANR_st_EGSM1EcoBtnSts)
  Data Type Conversion180/1 -> HCU/98(pCANR_st_EGSM1SBW1LvlPstn)
  Data Type Conversion179/1 -> HCU/101(pCANR_kmph_ABS1WhlSpdFL)
  Data Type Conversion178/1 -> HCU/102(pCANR_kmph_ABS1WhlSpdFR)
  Data Type Conversion186/1 -> HCU/103(pCANR_kmph_ABS1VehSpd)
  Data Type Conversion185/1 -> HCU/104(pCANR_kmph_ABS2WhlSpdRL)
  Data Type Conversion184/1 -> HCU/105(pCANR_kmph_ABS2WhlSpdRR)
  Data Type Conversion183/1 -> HCU/106(pCANR_bar_ABS2MasterCylPres)
  Data Type Conversion191/1 -> HCU/108(pCANR_bool_ABS3ABSErrSt)
  Data Type Conversion204/1 -> HCU/109(pCANR_bool_ABS3ABSIntv)
  Data Type Conversion203/1 -> HCU/110(pCANR_bool_ABS3ASRErrSt)
  Data Type Conversion202/1 -> HCU/111(pCANR_bool_ABS3ASRIntv)
  Data Type Conversion201/1 -> HCU/112(pCANR_bool_ABS3ESPErrSt)
  Data Type Conversion196/1 -> HCU/113(pCANR_bool_ABS3ESPIntv)
  Data Type Conversion195/1 -> HCU/114(pCANR_bool_ABS3HHCSt)
  Data Type Conversion194/1 -> HCU/115(pCANR_bool_ABS3HHCAvail)
  Data Type Conversion200/1 -> HCU/116(pCANR_Nm_ASR1TrqRdctFastASR1)
  Data Type Conversion199/1 -> HCU/117(pCANR_Nm_ASR1TrqIncrsMSR1)
  Data Type Conversion198/1 -> HCU/118(pCANR_bool_ASR1StTRFastASR1)
  Data Type Conversion197/1 -> HCU/119(pCANR_bool_ASR1StTIMSR1)
  Constant85/1 -> Data Type Conversion237/1
  Constant9/1 -> Data Type Conversion1/1
  Data Type Conversion1/1 -> HCU/99(pCANR_st_EGSM1SecBtnSt)
  Constant10/1 -> Data Type Conversion2/1
  Data Type Conversion2/1 -> HCU/100(pCANR_st_EGSM1ErrSt)
  Bus Selector29/4 -> Data Type Conversion31/1  "<ePARK_CAN_ERR>"
  Data Type Conversion31/1 -> HCU/85(pCANR_bool_EparkErrSt)
  Bus Selector/37 -> HCU_LeverInfo/1  "<HCU_LeverInfo>"
  In1/1 -> Bus Selector34/1, Bus Selector32/1, Bus Selector51/1, Bus Selector49/1, Bus Selector47/1, Bus Selector45/1, Bus Selector43/1, Bus Selector36/1, Bus Selector30/1, Bus Selector28/1, Bus Selector25/1, Bus Selector23/1, Bus Selector21/1, Bus Selector19/1, Bus Selector17/1, Bus Selector15/1, Bus Selector13/1, Bus Selector11/1, Bus Selector10/1, Bus Selector7/1, Bus Selector6/1, Bus Selector4/1, Bus Selector1/1
  Bus Selector49/1 -> Bus Selector50/1  "<IO>"
  Bus Selector50/1 -> Data Type Conversion238/1  "<SlowChrgSensr1Temp>"
  Bus Selector50/2 -> Data Type Conversion239/1  "<FastChrgSensr1Temp>"
  Bus Selector50/3 -> Data Type Conversion240/1  "<SlowChrgSensr2Temp>"
  Bus Selector50/4 -> Data Type Conversion241/1  "<FastChrgSensr2Temp>"
  Data Type Conversion32/1 -> HCU/62(pCANR_st_BMS5ChrgStationHandSt)
  Data Type Conversion39/1 -> HCU/124(pCANR_Nm_ABS6RegenTrqReq)
  Data Type Conversion38/1 -> HCU/123(pCANR_bool_ASR2StTIMSR2)
  Data Type Conversion40/1 -> HCU/125(pCANR_bool_ABS6StRegenTrqReq)
  Data Type Conversion35/1 -> HCU/120(pCANR_Nm_ASR2TrqRdctFastASR2)
  Data Type Conversion37/1 -> HCU/122(pCANR_bool_ASR2StTRFastASR2)
  Data Type Conversion36/1 -> HCU/121(pCANR_Nm_ASR2TrqIncrsMSR2)
  Data Type Conversion192/1 -> HCU/129(pCANR_bool_YRS1YRSErrSt)
  Data Type Conversion193/1 -> HCU/128(pCANR_bool_YRS1YRSSt)
  Data Type Conversion205/1 -> HCU/127(pCANR_mps2_YRS1AY1)
  Data Type Conversion206/1 -> HCU/126(pCANR_mps2_YRS1AX1)
  Data Type Conversion207/1 -> HCU/131(pCANR_mps2_YRS2AY1Ofst)
  Data Type Conversion208/1 -> HCU/130(pCANR_mps2_YRS2AX1Ofst)
  Data Type Conversion209/1 -> HCU/135(pCANR_bool_AC1ACCmprOnReq)
  Data Type Conversion210/1 -> HCU/136(pCANR_st_AC1ACSt)
  Data Type Conversion211/1 -> HCU/137(pCANR_st_AC1ACFanReq)
  Data Type Conversion212/1 -> HCU/138(pCANR_st_AC1PTCSt)
  Data Type Conversion3/1 -> HCU/132(pCANR_bool_Noise1OverVoltErr)
  Data Type Conversion4/1 -> HCU/133(pCANR_bool_Noise1UndrVoltErr)
  Data Type Conversion5/1 -> HCU/134(pCANR_bool_Noise1ShotCicutErr)
  Data Type Conversion10/1 -> HCU/150(pCANR_st_TBOX1InstnChrgReq)
  Data Type Conversion7/1 -> HCU/147(pCANR_st_TBOX1RemoteACReq)
  Data Type Conversion8/1 -> HCU/148(pCANR_st_TBOX1ChrgModeTbox)
  Data Type Conversion9/1 -> HCU/149(pCANR_st_TBOX1TimeChrgReq)
  Data Type Conversion217/1 -> HCU/144(pCANR_bool_ACInd)
  Data Type Conversion218/1 -> HCU/145(pCANR_st_ACIndBLWLvlInd)
  Data Type Conversion219/1 -> HCU/146(pCANR_degC_ACIndOutTempInd)
  Data Type Conversion6/1 -> HCU/143(pCANR_rpm_ACTestCmprSpd)
  Data Type Conversion213/1 -> HCU/139(pCANR_bool_AC1ACShtDwnEnblL)
  Data Type Conversion214/1 -> HCU/140(pCANR_w_AC1PwrCnsmpACL)
  Data Type Conversion215/1 -> HCU/141(pCANR_w_AC1PwrCnsmpACH)
  Data Type Conversion216/1 -> HCU/142(pCANR_bool_AC1ACShtDwnEnblH)
  Data Type Conversion11/1 -> HCU/151(pCANR_bool_TBOX1QueryReq)
  Data Type Conversion12/1 -> HCU/152(pCANR_st_TBOX1TboxSt)
  Data Type Conversion13/1 -> HCU/153(pCANR_na_TBOX2GPSYear)
  Data Type Conversion14/1 -> HCU/154(pCANR_na_TBOX2GPSMonth)
  Data Type Conversion15/1 -> HCU/155(pCANR_na_TBOX2GPSDay)
  Data Type Conversion16/1 -> HCU/156(pCANR_na_TBOX2GPSHour)
  Data Type Conversion17/1 -> HCU/157(pCANR_na_TBOX2GPSMinute)
  Data Type Conversion220/1 -> HCU/159(pCANR_st_ACC1ACCSt)
  Data Type Conversion221/1 -> HCU/160(pCANR_mps2_ACC1ACCDecelReq)
  Data Type Conversion222/1 -> HCU/161(pCANR_st_ACC1ACCStTrqReq)
  Data Type Conversion228/1 -> HCU/158(pCANR_st_ACC1ACCErrSt)
  Data Type Conversion18/1 -> HCU/168(pHWIN_mV_CruzSwt)
  Data Type Conversion19/1 -> HCU/169(pHWIN_mV_MCUWaterTemp)
  Data Type Conversion20/1 -> HCU/170(pHWIN_mV_AccPed1)
  Data Type Conversion21/1 -> HCU/171(pHWIN_mV_AccPed2)
  Data Type Conversion22/1 -> HCU/172(pHWIN_mV_VacPres)
  Data Type Conversion223/1 -> HCU/162(pCANR_Nm_ACC1ACCTrqReq)
  Data Type Conversion224/1 -> HCU/163(pCANR_st_ACC1ACCStACCDecelReq)
  Data Type Conversion225/1 -> HCU/164(pHWIN_mV_SlowChrgCnfrm)
  Data Type Conversion226/1 -> HCU/165(pHWIN_mV_FastChrgCnfrm)
  Data Type Conversion227/1 -> HCU/166(pHWIN_mV_IntlkA)
  Data Type Conversion229/1 -> HCU/167(pHWIN_mV_IntlkB)
  Data Type Conversion23/1 -> HCU/173(pHWIN_mV_BatVolt)
  Data Type Conversion237/1 -> HCU/185(pHWIN_st_EPark)
  Data Type Conversion238/1 -> HCU/181(pHWIN_degC_SlowChrgSensr1Temp)
  Data Type Conversion239/1 -> HCU/182(pHWIN_degC_FastChrgSensr1Temp)
  Data Type Conversion24/1 -> HCU/174(pHWIN_st_IMMO)
  Data Type Conversion240/1 -> HCU/183(pHWIN_degC_SlowChrgSensr2Temp)
  Data Type Conversion241/1 -> HCU/184(pHWIN_degC_FastChrgSensr2Temp)
  Data Type Conversion25/1 -> HCU/175(pHWIN_st_NoCANMsgRx)
  Data Type Conversion26/1 -> HCU/176(pHWIN_bool_KeyOn)
  Data Type Conversion27/1 -> HCU/177(pHWIN_bool_KeyStart)
  Data Type Conversion28/1 -> HCU/178(pHWIN_bool_MainBrkSt)
  Data Type Conversion29/1 -> HCU/179(pHWIN_bool_AssistBrkSt)
  Data Type Conversion30/1 -> HCU/180(pHWIN_bool_ECOSwt)
  Data Type Conversion33/1 -> HCU/187(s_DcDcBswErr_na)
  Data Type Conversion34/1 -> HCU/188(s_MotCtlrBswErr_na)
  Data Type Conversion60/1 -> HCU/189(s_ChrgrBswErr_na)
  Data Type Conversion61/1 -> HCU/190(s_ThermBswErr_na)
  Data Type Conversion62/1 -> HCU/191(s_BmsBswErr_na)
  Data Type Conversion63/1 -> HCU/192(s_ShftLvrBswErr_na)
  Data Type Conversion64/1 -> HCU/193(s_AirBagBswErr_na)
  Data Type Conversion65/1 -> HCU/194(s_EpsBswErr_na)
  Data Type Conversion66/1 -> HCU/195(s_IcBswErr_na)
  Data Type Conversion67/1 -> HCU/196(s_BcmBswErr_na)
  Data Type Conversion68/1 -> HCU/197(s_HmiBswErr_na)
  Data Type Conversion69/1 -> HCU/198(s_VacPmpBswErr_na)
  Data Type Conversion70/1 -> HCU/199(s_PwrBswErr_na)
  Data Type Conversion71/1 -> HCU/200(s_VirtIgBswErr_na)
  Data Type Conversion72/1 -> HCU/201(s_PrkgLockBswErr_na)
  Data Type Conversion73/1 -> HCU/202(s_PrkgLockErrSts_na)
  Data Type Conversion74/1 -> HCU/203(s_HvBswErr_na)
  Data Type Conversion75/1 -> HCU/204(s_TBoxBswErr_na)
  Data Type Conversion76/1 -> HCU/205(s_ChrgSnsrBswErr_na)
  Data Type Conversion77/1 -> HCU/206(s_MotBatEmgcySignalErr_na)
  Data Type Conversion78/1 -> HCU/207(s_EEMBswErr_na)
  Data Type Conversion79/1 -> HCU/208(s_NoiseSimuBswErr_na)
  Data Type Conversion80/1 -> HCU/209(s_PasvStaCheckBswErr_na)
  Data Type Conversion82/1 -> HCU/210(s_PEPSBswErr_na)
  HCU/1(pOUTP_st_ACU1Crash) -> [pOUTP_st_Airbag1CrashIntsy]
  HCU/2(pOUTP_st_HCU2ChrgHeatPms) -> [pOUTP_st_HCU2ChrgrHeatReq]
  HCU/3(pOUTP_st_HCU2ChrgConnSt) -> [s_ChrgrPlgSwt_na]
  HCU/4(pOUTP_bool_HCU2MainPlusCtrl) -> [s_MaiPosContCmd_na]
  HCU/5(pOUTP_bool_HCU2MainMinusCtrl) -> [s_MaiNegContCmd_na]
  HCU/6(pOUTP_bool_HCU2PreChrgCtrl) -> [s_MaiPrecContCmd_na]
  HCU/7(pOUTP_bool_HCU2ChrgPlusCtrl) -> [pOUTP_bool_HCU2ChrgPlusCtrl]
  HCU/8(pOUTP_bool_HCU2ChrgMinusCtrl) -> [pOUTP_bool_HCU2ChrgMinusCtrl]
  HCU/9(pOUTP_bool_HCU2ChrgPms) -> [s_BatChrgPerm_na]
  HCU/10(pOUTP_bool_HCU2SleepIndSig) -> [s_CanSlpCmd_na]
  HCU/11(pOUTP_V_HCU2DCDCOutVoltReq) -> [s_DcDcOutUSp_V]
  HCU/12(pOUTP_bool_HCU2DCDCEnbl) -> [e_DcDcCmd_na]
  HCU/13(pOUTP_st_HCU2VehOprtMode) -> [pOUTP_st_HCU2VehOprtMode]
  HCU/14(pOUTP_Nm_HCU3TMTrqReqMCU1) -> [pOUTP_Nm_HCU3TMTorqReqToMCU1]
  HCU/15(pOUTP_bool_HCU3RapidDisChrgMCU1) -> [pOUTP_bool_HCU3MotRpdDchaReqToMCU1]
  HCU/16(pOUTP_st_HCU3StTMReqMCU1) -> [pOUTP_bool_HCU3MotCtlrStModReqToMCU1]
  HCU/17(pOUTP_bool_AntijerkDisblMCU1) -> [pOUTP_bool_HCU3AntijerkOffReqToMCU1]
  HCU/18(pOUTP_bool_HCU3StopReqMCU1) -> [pOUTP_bool_HCU3StopReqToMCU1]
  HCU/19(pOUTP_Nm_HCU3TMTrqReqMCU2) -> [pOUTP_Nm_HCU5TMToqReqToMCU2]
  HCU/20(pOUTP_bool_HCU3RapidDisChrgMCU2) -> [pOUTP_bool_HCU5MotRpdDchaReqToMCU2]
  HCU/26(pOUTP_st_HCU10ChrgrSt) -> [pOUTP_st_HCU10ChrgSt]
  HCU/21(pOUTP_st_HCU3StTMReqMCU2) -> [pOUTP_bool_HCU5MotCtlrStModReqToMCU2]
  HCU/22(pOUTP_bool_AntijerkDisblMCU2) -> [pOUTP_bool_HCU5AntijerkOffReqToMCU2]
  HCU/23(pOUTP_bool_HCU3StopReqMCU2) -> [pOUTP_bool_HCU5StopReqToMCU2]
  HCU/24(pOUTP_kmph_HCU4VehSpdABS) -> [pOUTP_kmph_HCU4VehSpd]
  HCU/25(pOUTP_V_HCU10BatPackVolt) -> [pOUTP_V_HCU10BatVoltHigh]
  HCU/27(pOUTP_A_HCU10BatPackCurr) -> [pOUTP_A_HCU10BatCurr]
  HCU/28(pOUTP_st_HCU10IslaWarn) -> [pOUTP_st_HCU10IslaWarning]
  HCU/29(pOUTP_pct_HCU10BatPackSOC) -> [pOUTP_pct_HCU10BatSOC]
  HCU/30(pOUTP_degC_HCU10BatPackTemp) -> [pOUTP_degC_HCU10BatTemp]
  HCU/31(pOUTP_pct_HCU10OutPwrPct) -> [pOUTP_pct_HCU10OutPwr]
  HCU/32(pOUTP_st_HCU10DCDCSt) -> [pOUTP_st_HCU10DCDCSt]
  HCU/33(pOUTP_bool_HCU10IntlkSysFlt) -> [pOUTP_bool_HCU10IntlkSysFlt]
  HCU/34(pOUTP_bool_HCU10SleepIndSig) -> [pOUTP_bool_HCU10SleepIndSig]
  HCU/35(pOUTP_bool_HCU10ECOSwtInd) -> [pOUTP_bool_HCU10ECOSwtInd]
  HCU/36(pOUTP_kw_HCU13InstnsPwrCnsmp) -> [pOUTP_kw_HCU13InstnsPwrCnsmp]
  HCU/37(pOUTP_min_HCU13RemainChrgTime) -> [pOUTP_s_HCU13RemainChrgTime]
  HCU/38(pOUTP_km_HCU13RemainDrvDist) -> [s_RemainDrvgRng_km]
  HCU/39(pOUTP_st_HCU13BatHeatSt) -> [pOUTP_st_HCU13BatHeatDsply]
  HCU/40(pOUTP_st_HCU13ChrgConnSt) -> [pOUTP_st_HCU13ChrgConnSt]
  HCU/42(pOUTP_bool_HCU13TMErrSt) -> [pOUTP_bool_HCU13TMFlt]
  HCU/43(pOUTP_bool_HCU13TMTempWarn) -> [pOUTP_bool_HCU13TMTempHighAlart]
  HCU/41(pHMI_bool_BatteryError) -> [pOUTP_bool_HCU13BatErr]
  HCU/46(pOUTP_bool_HCU13ACPTCCnfig) -> [pOUTP_bool_HCU13ACPTCCnfig]
  HCU/47(pOUTP_st_HCU13BatPackCoolReq) -> [s_BatCoolgReq_na]
  HCU/44(pOUTP_st_HCU13IGKeyPstn) -> [pOUTP_st_HCU13IgnKeyPos]
  HCU/48(pOUTP_bool_HCU13IGOffReq) -> [HCU_IGOFFRequest]
  HCU/49(pHMI_bool_HCU13BatSOCLowAlart) -> [HCU_BatterySOCWarning]
  HCU/50(pOUTP_bool_HCU13BatTempWarn) -> [HCU_BatteryPackTempWarning]
  HCU/51(pOUTP_bool_HCU13RemanACOnTip) -> [HCU_RemainACOnTip]
  HCU/52(pOUTP_st_HCU13NoiseVoiceCnfig) -> [HCU_NoiseSimuVoiceConfig]
  HCU/53(pOUTP_st_HCU14LvlInfo) -> [HCU_LeverInfo]
  HCU/54(pOUTP_pct_HCU4AccelPedPstn) -> [HCU_AccPedPosition]
  HCU/57(pOUTP_st_HCU4BrkSwt) -> [HCU_BrakeSwitch]
  HCU/55(pOUTP_pct_HCU4CalcAccelPedPstn) -> [HCU_CalcAccPedPos]
  HCU/56(pOUTP_bool_HCU4KickDwnReq) -> [HCU_KickdownRequest]
  HCU/58(pOUTP_bool_HCU4ACOnFeedBack) -> [HCU_ACOnFeedback]
  HCU/59(pOUTP_st_HCU4CruzCtrlSt) -> [HCU_CrsCtlSts]
  HCU/60(pOUTP_bool_HCU4AccelPedOvrid) -> [HCU_AccPedOverride]
  HCU/63(pOUTP_st_HCU5VehOprtMode) -> [pOUTP_st_HCU5VehOprtMode]
  HCU/64(pOUTP_st_HCU5EVReady) -> [pOUTP_st_HCU5EVReady]
  HCU/65(pOUTP_st_HCU5HCUStatus) -> [pOUTP_st_HCU5HCUStatus]
  HCU/67(pOUTP_kmph_HCU8CrsSpdSetPnt) -> [HCU_CCTargetSpeed]
  HCU/68(pOUTP_bool_HCU8RespACC) -> [HCU_ResponseACC]
  HCU/69(pOUTP_bool_HCU8CCMainSwt) -> [HCU_CCMainSwitch]
  HCU/70(pOUTP_bool_HCU8CCCancelSwt) -> [HCU_CCCancelSwitch]
  HCU/71(pOUTP_bool_HCU8CCSetOrCoastSwt) -> [HCU_CCSetOfCoastSwitch]
  HCU/74(pOUTP_bool_HCU8CCRsmOrAccelSwt) -> [HCUCCResumeOrAccSwitch]
  HCU/72(pOUTP_bool_HCU8HeadwaySwt) -> [HCU_HeadWaySwitch]
  HCU/73(pOUTP_bool_HCU8CCSwtErr) -> [HCU_CCSwitchError]
  HCU/75(pOUTP_st_HCUEparkPrkReq) -> [HCU_ParkRequest]
  HCU/76(pOUTP_Nm_HCU15ActTrq) -> [pOUTP_Nm_HCU15ActTrq]
  HCU/77(pOUTP_Nm_HCU15MAMTrq) -> [pOUTP_Nm_HCU15MAMTrq]
  HCU/86(pOUTP_pwm_PTCPWMCtrl) -> [s_PtcCtrlCmd_p100]
  HCU/87(pOUTP_bool_RadorValve1Ctrl1) -> [pOUTP_bool_RadorValveCtrlB]
  HCU/88(pOUTP_bool_RadorValve1Ctrl2) -> [pOUTP_bool_RadorValveCtrlC]
  HCU/89(pOUTP_bool_BatPTCValve2Ctrl1) -> [pOUTP_bool_BatPTCValveCtrlB]
  HCU/90(pOUTP_bool_BatPTCValve2Ctrl2) -> [pOUTP_bool_BatPTCValveCtrlC]
  HCU/91(pOUTP_bool_VacPmpRlyCtrl) -> [s_BrkVacPmpCmd_p100]
  HCU/92(pOUTP_bool_LoCoolFanRlyCtrl) -> [s_LoSpdFanCmd_na]
  HCU/93(pOUTP_bool_HiCoolFanRlyCtrl) -> [s_HiSpdFanCmd_na]
  HCU/94(pOUTP_pwm_MotWaterPump1Ctrl) -> [s_MotWtrPmpCmd_p100]
  HCU/95(pOUTP_pwm_BatWaterPumpCtrl) -> [s_BatWtrPmpCmd_p100]
  HCU/96(pOUTP_bool_MCUVirtIgOn) -> [s_MotVirtIgOn_na]
  HCU/97(pOUTP_bool_MainRlyCtrl) -> [s_MaiRlyCtlCmd_na]
  HCU/98(pOUTP_bool_VCUSleep) -> [pOUTP_bool_VCUSleep]
  HCU/99(pOUTP_pwm_MotWaterPump2Ctrl) -> [IO_Mot2WtrPmpCmd]
  Bus Selector39/1 -> Bus Selector40/1  "<YRS>"
  Bus Selector51/1 -> Bus Selector52/1  "<ESP>"
  Bus Selector52/5 -> Data Type Conversion39/1  "<ABS6RegenTrqReq>"
  Bus Selector52/4 -> Data Type Conversion38/1  "<ASR2StTIMSR2>"
  Bus Selector52/2 -> Data Type Conversion36/1  "<ASR2TrqIncrsMSR2>"
  Bus Selector52/1 -> Data Type Conversion35/1  "<ASR2TrqRdctFastASR2>"
  Bus Selector52/6 -> Data Type Conversion40/1  "<ABS6StRegenTrqReq>"
  Bus Selector52/3 -> Data Type Conversion37/1  "<ASR2StTRFastASR2>"
  HCU/78(pOUTP_Nm_HCU18MCU1ActTMTrq) -> [pOUTP_Nm_HCU18MCU1ActTMTrq]
  HCU/79(pOUTP_Nm_HCU18MCU1MAMTrq) -> [pOUTP_Nm_HCU18MCU1MAMTrq]
  HCU/80(pOUTP_Nm_HCU18MCU1MAGTrq) -> [pOUTP_Nm_HCU18MCU1MAGTrq]
  HCU/82(pOUTP_Nm_HCU19MCU2ActTMTrq) -> [pOUTP_Nm_HCU19MCU2ActTMTrq]
  HCU/83(pOUTP_Nm_HCU19MCU2MAMTrq) -> [pOUTP_Nm_HCU19MCU2MAMTrq]
  HCU/84(pOUTP_Nm_HCU19MCU2MAGTrq) -> [pOUTP_Nm_HCU19MCU2MAGTrq]
  [pOUTP_Nm_HCU15ActTrq] -> Bus Creator14/1  "HCU15ActTrq"
  [pOUTP_Nm_HCU15MAMTrq] -> Bus Creator14/2  "HCU15MAMTrq"
  [pOUTP_Nm_HCU15IndicateDrvTrq] -> Bus Creator14/3  "HCU15IndicateDrvTrq"
  Bus Creator14/1 -> [PT_HCU_15]
  [pOUTP_Nm_HCU18MCU1ActTMTrq] -> Bus Creator15/1  "HCU18MCU1ActTMTrq"
  [pOUTP_Nm_HCU18MCU1MAMTrq] -> Bus Creator15/2  "HCU18MCU1MAMTrq"
  [pOUTP_Nm_HCU18MCU1MAGTrq] -> Bus Creator15/3  "HCU18MCU1MAGTrq"
  Bus Creator15/1 -> [PT_HCU_18]
  [pOUTP_Nm_HCU19MCU2ActTMTrq] -> Bus Creator20/1  "HCU19MCU2ActTMTrq"
  [pOUTP_Nm_HCU19MCU2MAMTrq] -> Bus Creator20/2  "HCU19MCU2MAMTrq"
  [pOUTP_Nm_HCU19MCU2MAGTrq] -> Bus Creator20/3  "HCU19MCU2MAGTrq"
  Bus Creator20/1 -> [PT_HCU_19]
  [PT_HCU_15] -> Bus Creator18/8  "PT_HCU_15"
  [PT_HCU_18] -> Bus Creator18/9  "PT_HCU_18"
  [PT_HCU_19] -> Bus Creator18/10  "PT_HCU_19"
  Bus Selector/42 -> PT_HCU_8/1  "<PT_HCU_8>"
  Bus Selector/41 -> PT_HCU_4/1  "<PT_HCU_4>"
  Bus Selector/38 -> PT_HCU_15/1  "<PT_HCU_15>"
  Bus Selector/40 -> PT_HCU_19/1  "<PT_HCU_19>"
  Bus Selector/39 -> PT_HCU_18/1  "<PT_HCU_18>"
  Data Type Conversion147/1 -> HCU/7(pCANR_st_MCU11TMErrSt)
  Data Type Conversion148/1 -> HCU/6(pCANR_st_MCU11TMSt)
  Data Type Conversion149/1 -> HCU/5(pCANR_bool_MCU11PreChrgAllow)
  Data Type Conversion151/1 -> HCU/4(pCANR_bool_MCU11TMTrqValid)
  Data Type Conversion150/1 -> HCU/2(pCANR_Nm_MCU11TMTrq)
  Data Type Conversion152/1 -> HCU/3(pCANR_V_MCU11TMCapVolt)
  Data Type Conversion153/1 -> HCU/1(pCANR_rpm_MCU11TMSpd)
  Bus Selector2/8 -> Data Type Conversion41/1  "<MCU1_ShutdownEnable>"
  Data Type Conversion41/1 -> HCU/8(pCANR_bool_MCU11ShtdwnAllow)
  Data Type Conversion140/1 -> HCU/15(pCANR_st_MCU21TMErrSt)
  Data Type Conversion143/1 -> HCU/12(pCANR_bool_MCU21TMTrqValid)
  Data Type Conversion141/1 -> HCU/14(pCANR_st_MCU21TMSt)
  Data Type Conversion142/1 -> HCU/13(pCANR_bool_MCU21PreChrgAllow)
  Data Type Conversion144/1 -> HCU/11(pCANR_V_MCU21TMCapVolt)
  Data Type Conversion145/1 -> HCU/10(pCANR_Nm_MCU21TMTrq)
  Data Type Conversion146/1 -> HCU/9(pCANR_rpm_MCU21TMSpd)
  Bus Selector3/8 -> Data Type Conversion42/1  "<MCUShutdownEnable>"
  Data Type Conversion42/1 -> HCU/16(pCANR_bool_MCU21ShtdwnAllow)
  Bus Selector48/4 -> Data Type Conversion229/1  "<InterlockB (signal 3)>"
  Bus Selector48/3 -> Data Type Conversion227/1  "<interlockA (signal 2)>"
  HCU/45(pOUTP_st_HCU13VehDeiceHeatPmt) -> [HCU_VehicleDeiceHeatPermit]
  Data Type Conversion156/1 -> HCU/76(pCANR_st_EPS1EPSErrSt)
  Constant15/1 -> Data Type Conversion43/1
  Data Type Conversion43/1 -> HCU/75(pCANR_st_ACU1DrvSideBuckSts)
  Constant19/1 -> Data Type Conversion44/1
  Data Type Conversion44/1 -> HCU/107(pCANR_pct_ABS2BrakePedalPos)
  Constant23/1 -> Product/2
  Product/1 -> Saturation/1
  Lookup Table/1 -> HCU/186(pHWIN_mV_VacAmbientPres)
  Constant24/1 -> Product/1
  Saturation/1 -> Lookup Table/1
